simulink model "gm_sampleModel1492_sub"  (R2023a)
settings: Solver=VariableStepAuto  StartTime=0.0  StopTime=10.0  RelTol=1e-3
libraries: hdlsllib x2, simulink x1
settings Model: Creator=user1  LastModifiedBy=user1
settings OptimizationCC: BlockReduction=off  ConditionallyExecuteInputs=off
settings DebuggingCC: InheritedTsInSrcMsg=none

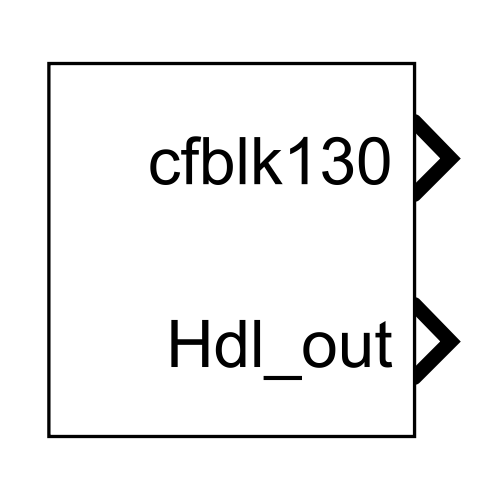
[thumbnail: Simulink's stored preview of the top-level diagram]
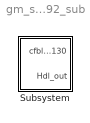
== system gm_sampleModel1492_sub ==
  Subsystem : Subsystem

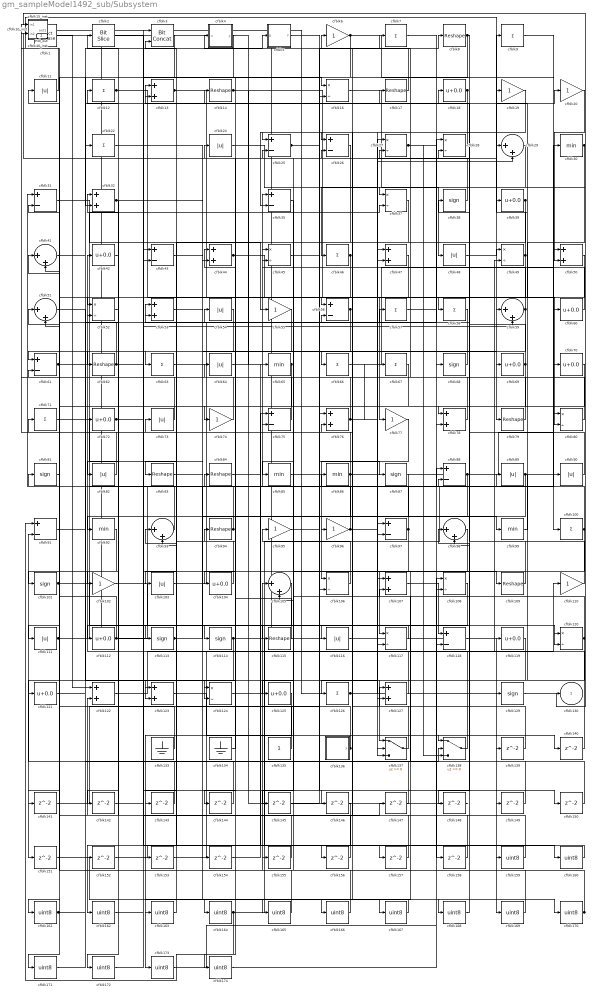
== system gm_sampleModel1492_sub/Subsystem ==
  cfblk1 : simulink/Logic and Bit Operations/Detect Decrease  vinit=0.0  OutDataTypeStr=uint8
      settings: LibrarySourceBlock=|
      | hdlsllib/Logic and Bit
      | Operations/Detect
      | Decrease
  cfblk{7,9,12,22,46,57..58,63,66..67,71,100,126} (13 alike) : Sum  Inputs=+  OutDataTypeStr=uint8
  cfblk{38,68,81,87,101,113..114,129} (8 alike) : Signum
  cfblk{6,19..20,55,74,77,95..96,102,110} (10 alike) : Gain  OutDataTypeStr=uint8
  cfblk{11,24,48,54,64,73,82,89..90,103,111,116} (12 alike) : Abs  OutDataTypeStr=uint8  SaturateOnIntegerOverflow=off
  cfblk{18,39,42,60,69..70,72,104,112,119,121,125} (12 alike) : Bias  Bias=0.0  SaturateOnIntegerOverflow=off
  cfblk{29,41,51,59,93,98,105} (7 alike) : Sum  Inputs=|++  OutDataTypeStr=uint8
  cfblk{16,27..28,37,45,49,52,80,106,108,117,120,124} (13 alike) : Product  Inputs=*/  OutDataTypeStr=uint8  RndMeth=Zero  SaturateOnIntegerOverflow=on
  cfblk{13,32,44,47,50,53,76,78,107,122..123,127} (12 alike) : Sum  OutDataTypeStr=uint8
  cfblk{8,14,17,62,79,83..84,94,109,115} (10 alike) : Reshape
  cfblk10_inst : Subsystem
  cfblk{25..26,31,35,43,56,61,75,88,91,97,118} (12 alike) : Sum  Inputs=+-  OutDataTypeStr=uint8
  cfblk133 : Ground
  cfblk134 : Ground
  cfblk135 : Constant  OutDataTypeStr=uint8  SampleTime=-1
  cfblk136 : Subsystem  mask(Counter Limited){uplimit=double(7), tsamp=double(-1)}
      mask prompts: uplimit "Simulink:masks:UpperLimit_MP"; tsamp "Simulink:masks:SampleTime_MP"
      mask help: Simulink:masks:CounterLimited_MD
      mask init:
      | nbits = double(8);
      | tsamp = double(-1);
      | uplimit = double(7);
  cfblk137 : Switch  OutDataTypeStr=uint8  SaturateOnIntegerOverflow=off  InputSameDT=off
  cfblk138 : Switch  OutDataTypeStr=uint8  SaturateOnIntegerOverflow=off  InputSameDT=off
  cfblk{139..158} (20 alike) : Delay  SampleTime=1
  cfblk{159..174} (16 alike) : DataTypeConversion  OutDataTypeStr=uint8  SaturateOnIntegerOverflow=off  RndMeth=Floor
  cfblk15_inst : Subsystem
  cfblk2 : hdlsllib/Logic and Bit Operations/Bit Slice  lidx=7  ridx=0
  cfblk3 : hdlsllib/Logic and Bit Operations/Bit Concat  numInputs=2
  cfblk{30,65,85..86,92,99} (6 alike) : MinMax  OutDataTypeStr=uint8
  cfblk4 : Subsystem  mask(Compare To Zero){relop=<=, OutDataTypeStr=uint8, ZeroCross=on}
      mask prompts: relop "Simulink:masks:Operator_MP"; OutDataTypeStr "Simulink:masks:OutputDataType_MP"; ZeroCross "Simulink:masks:EnableZerocrossingDetection_MP"
      mask help: Simulink:masks:CompareToZero_MD
      mask init:
      | OutDataTypeStr = 'uint8';
      | ZeroCross = 'on';
      | blkName = 'sampleModel1492_sub/Subsystem/cfblk4';
      | relop = '<=';
      | setValue = 'fixdt(0, 8)';
      mask TypeOptions relop: == | ~= | < | <= | >= | >
      mask TypeOptions OutDataTypeStr: Simulink:masks:uint8 | Simulink:masks:boolean
      mask Callback ZeroCross: sl('zeroCrossEnable', gcbh);
      mask Display: disp([relop,' 0'])
  cfblk40_inst : Subsystem
  cfblk5 : Subsystem  mask(Detect Fall Nonpositive){vinit=double(0), InputProcessing=Elements as channels (sample based), OutDataTypeStr=uint8}
      mask prompts: vinit "Simulink:masks:InitialCondition_MP"; InputProcessing "Simulink:masks:InputProcessing_MP"; OutDataTypeStr "Simulink:masks:OutputDataType_MP"
      mask help: Simulink:masks:DetectFallNonpositive_MD
      mask init:
      | InputProcessing = 'Elements as channels (sample based)';
      | OutDataTypeStr = 'uint8';
      | vinit = double(0);
      mask TypeOptions InputProcessing: Simulink:masks:ColumnsAsChannelsFrameBased | Simulink:masks:ElementsAsChannelsSampleBased
      mask TypeOptions OutDataTypeStr: Simulink:masks:uint8 | Simulink:masks:boolean
      mask Display: fprintf('U <= 0\n&  NOT\nU/z <= 0')
  cfblk130 : Outport  OutDataTypeStr=uint8  SampleTime=1  VectorParamsAs1DForOutWhenUnconnected=off
  Hdl_out : Outport  Port=2  OutDataTypeStr=uint8  SampleTime=1
  wires:
  cfblk1/1 -> cfblk122/1
  cfblk10_inst/1(out1) -> cfblk90/1
  cfblk100/1 -> cfblk81/1, cfblk35/1, cfblk117/1
  cfblk101/1 -> cfblk116/1, cfblk120/2
  cfblk102/1 -> cfblk114/1
  cfblk103/1 -> cfblk56/2
  cfblk104/1 -> cfblk73/1
  cfblk105/1 -> cfblk164/1
  cfblk106/1 -> cfblk95/1
  cfblk107/1 -> cfblk118/1
  cfblk108/1 -> cfblk172/1
  cfblk109/1 -> cfblk13/1
  cfblk11/1 -> cfblk79/1
  cfblk110/1 -> cfblk53/1
  cfblk111/1 -> cfblk84/1, cfblk37/2
  cfblk112/1 -> cfblk88/2, cfblk11/1
  cfblk113/1 -> cfblk88/1, Hdl_out/1
  cfblk114/1 -> cfblk160/1, cfblk123/2, cfblk151/1
  cfblk115/1 -> cfblk54/1
  cfblk116/1 -> cfblk107/1
  cfblk117/1 -> cfblk113/1
  cfblk118/1 -> cfblk169/1
  cfblk119/1 -> cfblk137/1
  cfblk12/1 -> cfblk80/2, cfblk16/1
  cfblk120/1 -> cfblk45/1, cfblk126/1
  cfblk121/1 -> cfblk5/1(U)
  cfblk122/1 -> cfblk110/1
  cfblk123/1 -> cfblk138/1
  cfblk124/1 -> cfblk140/1
  cfblk125/1 -> cfblk173/1
  cfblk126/1 -> cfblk47/2, cfblk6/1
  cfblk127/1 -> cfblk75/2
  cfblk129/1 -> cfblk10_inst/1(in1)
  cfblk13/1 -> cfblk158/1, cfblk117/2
  cfblk133/1 -> cfblk51/1
  cfblk134/1 -> cfblk44/1
  cfblk135/1 -> cfblk94/1
  cfblk136/1(y) -> cfblk24/1, cfblk13/2
  cfblk137/1 -> cfblk76/2
  cfblk138/1 -> cfblk42/1
  cfblk139/1 -> cfblk127/1
  cfblk14/1 -> cfblk60/1, cfblk65/1
  cfblk140/1 -> cfblk47/1
  cfblk141/1 -> cfblk16/2
  cfblk142/1 -> cfblk43/2
  cfblk143/1 -> cfblk91/2
  cfblk144/1 -> cfblk52/2
  cfblk145/1 -> cfblk76/1
  cfblk146/1 -> cfblk162/1
  cfblk147/1 -> cfblk53/2
  cfblk148/1 -> cfblk1/1
  cfblk149/1 -> cfblk107/2
  cfblk15_inst/1(out1) -> cfblk119/1
  cfblk150/1 -> cfblk93/1
  cfblk151/1 -> cfblk168/1
  cfblk152/1 -> cfblk159/1
  cfblk153/1 -> cfblk49/2
  cfblk154/1 -> cfblk75/1
  cfblk155/1 -> cfblk122/2
  cfblk156/1 -> cfblk32/1
  cfblk157/1 -> cfblk41/2
  cfblk158/1 -> cfblk2/1
  cfblk159/1 -> cfblk26/2
  cfblk16/1 -> cfblk48/1
  cfblk160/1 -> cfblk152/1
  cfblk161/1 -> cfblk18/1, cfblk138/2
  cfblk162/1 -> cfblk3/1
  cfblk163/1 -> cfblk3/2
  cfblk164/1 -> cfblk91/1, cfblk80/1
  cfblk165/1 -> cfblk105/1
  cfblk166/1 -> cfblk105/2
  cfblk167/1 -> cfblk163/1
  cfblk168/1 -> cfblk98/1
  cfblk169/1 -> cfblk98/2
  cfblk17/1 -> cfblk4/1(u)
  cfblk170/1 -> cfblk155/1, cfblk71/1
  cfblk171/1 -> cfblk22/1
  cfblk172/1 -> cfblk147/1
  cfblk173/1 -> cfblk108/1
  cfblk174/1 -> cfblk108/2
  cfblk18/1 -> cfblk35/2, cfblk166/1, cfblk137/3
  cfblk19/1 -> cfblk26/1
  cfblk2/1 -> cfblk109/1
  cfblk20/1 -> cfblk50/2
  cfblk22/1 -> cfblk170/1
  cfblk24/1 -> cfblk97/1
  cfblk25/1 -> cfblk87/1, cfblk58/1
  cfblk26/1 -> cfblk93/2
  cfblk27/1 -> cfblk68/1, cfblk138/3
  cfblk28/1 -> cfblk25/1
  cfblk29/1 -> cfblk46/1
  cfblk3/1 -> cfblk161/1
  cfblk30/1 -> cfblk59/1, cfblk37/1
  cfblk31/1 -> cfblk55/1
  cfblk32/1 -> cfblk44/2, cfblk112/1
  cfblk35/1 -> cfblk115/1
  cfblk37/1 -> cfblk145/1
  cfblk38/1 -> cfblk15_inst/2(in2)
  cfblk39/1 -> cfblk123/1, cfblk74/1
  cfblk4/1(y) -> cfblk32/2
  cfblk40_inst/1(out1) -> cfblk130/1
  cfblk41/1 -> cfblk17/1
  cfblk42/1 -> cfblk82/1
  cfblk43/1 -> cfblk69/1
  cfblk44/1 -> cfblk97/2, cfblk77/1
  cfblk45/1 -> cfblk8/1
  cfblk46/1 -> cfblk111/1, cfblk45/2, cfblk144/1
  cfblk47/1 -> cfblk63/1
  cfblk48/1 -> cfblk49/1
  cfblk49/1 -> cfblk118/2, cfblk9/1
  cfblk5/1(Y) -> cfblk150/1
  cfblk50/1 -> cfblk52/1
  cfblk51/1 -> cfblk127/2
  cfblk52/1 -> cfblk92/1
  cfblk53/1 -> cfblk99/1
  cfblk54/1 -> cfblk171/1
  cfblk55/1 -> cfblk143/1
  cfblk56/1 -> cfblk83/1, cfblk124/2
  cfblk57/1 -> cfblk120/1
  cfblk58/1 -> cfblk85/1
  cfblk59/1 -> cfblk78/1, cfblk56/1, cfblk25/2
  cfblk6/1 -> cfblk70/1, cfblk61/1
  cfblk60/1 -> cfblk39/1
  cfblk61/1 -> cfblk121/1, cfblk28/1
  cfblk62/1 -> cfblk14/1, cfblk10_inst/2(in2), cfblk149/1
  cfblk63/1 -> cfblk27/1
  cfblk64/1 -> cfblk157/1
  cfblk65/1 -> cfblk141/1, cfblk124/1
  cfblk66/1 -> cfblk30/1
  cfblk67/1 -> cfblk142/1
  cfblk68/1 -> cfblk62/1
  cfblk69/1 -> cfblk78/2, cfblk104/1, cfblk28/2, cfblk66/1
  cfblk7/1 -> cfblk139/1
  cfblk70/1 -> cfblk153/1
  cfblk71/1 -> cfblk154/1
  cfblk72/1 -> cfblk59/2, cfblk20/1, cfblk156/1
  cfblk73/1 -> cfblk41/1
  cfblk74/1 -> cfblk15_inst/1(in1)
  cfblk75/1 -> cfblk43/1
  cfblk76/1 -> cfblk31/2, cfblk29/2, cfblk67/1
  cfblk77/1 -> cfblk106/1
  cfblk78/1 -> cfblk64/1
  cfblk79/1 -> cfblk7/1
  cfblk8/1 -> cfblk174/1, cfblk148/1
  cfblk80/1 -> cfblk27/2
  cfblk81/1 -> cfblk51/2
  cfblk82/1 -> cfblk40_inst/1(in1)
  cfblk83/1 -> cfblk165/1
  cfblk84/1 -> cfblk146/1
  cfblk85/1 -> cfblk106/2
  cfblk86/1 -> cfblk40_inst/2(in2), cfblk102/1
  cfblk87/1 -> cfblk96/1
  cfblk88/1 -> cfblk50/1, cfblk103/1
  cfblk89/1 -> cfblk137/2, cfblk129/1
  cfblk9/1 -> cfblk100/1
  cfblk90/1 -> cfblk38/1
  cfblk91/1 -> cfblk57/1
  cfblk92/1 -> cfblk101/1
  cfblk93/1 -> cfblk12/1
  cfblk94/1 -> cfblk61/2, cfblk31/1
  cfblk95/1 -> cfblk89/1
  cfblk96/1 -> cfblk29/1, cfblk86/1
  cfblk97/1 -> cfblk72/1, cfblk125/1
  cfblk98/1 -> cfblk167/1
  cfblk99/1 -> cfblk19/1

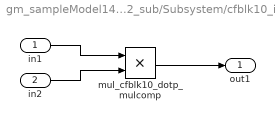
== system gm_sampleModel1492_sub/Subsystem/cfblk10_inst ==
  in1 : Inport  OutDataTypeStr=uint8  SampleTime=1
  in2 : Inport  Port=2  OutDataTypeStr=uint8  SampleTime=1
  mul_cfblk10_dotp_mulcomp : Product  Inputs=**  OutDataTypeStr=uint8  SampleTime=1
  out1 : Outport  OutDataTypeStr=uint8  SampleTime=1
  wires:
  in1/1 -> mul_cfblk10_dotp_mulcomp/1
  in2/1 -> mul_cfblk10_dotp_mulcomp/2
  mul_cfblk10_dotp_mulcomp/1 -> out1/1

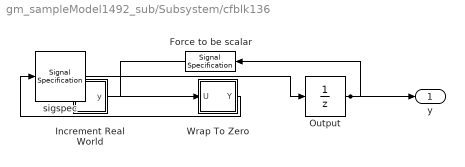
== system gm_sampleModel1492_sub/Subsystem/cfblk136 ==
  Force to be scalar : SignalSpecification  DisableCoverage=on  Dimensions=1
  Increment Real World : Subsystem  mask(Real World Value Increment){}
      mask help: Simulink:masks:RealWorldValueIncrement_MD
      mask Display: disp('V++')
  Output : UnitDelay  InitialCondition=0.0  SampleTime=tsamp  HasFrameUpgradeWarning=on
  Wrap To Zero : Subsystem  mask(Wrap To Zero){Threshold=double(7)}
      mask prompts: Threshold "Simulink:masks:Threshold_MP"
      mask help: Simulink:masks:WrapToZero_MD
  sigspec : SignalSpecification  OutDataTypeStr=uint8  Dimensions=1
  y : Outport  SampleTime=1
  wires:
  Force to be scalar/1 -> Increment Real World/1(u)
  Increment Real World/1(y) -> Wrap To Zero/1(U)
  Output/1 -> Force to be scalar/1, y/1
  Wrap To Zero/1(Y) -> sigspec/1
  sigspec/1 -> Output/1

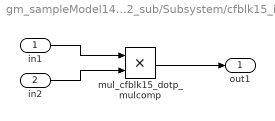
== system gm_sampleModel1492_sub/Subsystem/cfblk15_inst ==
  in1 : Inport  OutDataTypeStr=uint8  SampleTime=1
  in2 : Inport  Port=2  OutDataTypeStr=uint8  SampleTime=1
  mul_cfblk15_dotp_mulcomp : Product  Inputs=**  OutDataTypeStr=uint8  SampleTime=1
  out1 : Outport  OutDataTypeStr=uint8  SampleTime=1
  wires:
  in1/1 -> mul_cfblk15_dotp_mulcomp/1
  in2/1 -> mul_cfblk15_dotp_mulcomp/2
  mul_cfblk15_dotp_mulcomp/1 -> out1/1

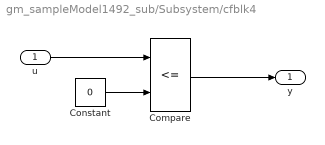
== system gm_sampleModel1492_sub/Subsystem/cfblk4 ==
  u : Inport  OutDataTypeStr=uint8  SampleTime=1
  Compare : RelationalOperator  Operator=<=  OutDataTypeStr=fixdt(0, 8)
  Constant : Constant  DisableCoverage=on  Value=0  OutDataTypeStr=Inherit: Inherit via back propagation  SampleTime=-1  PreserveConstantTs=on
  y : Outport  SampleTime=1
  wires:
  u/1 -> Compare/1
  Compare/1 -> y/1
  Constant/1 -> Compare/2

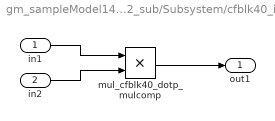
== system gm_sampleModel1492_sub/Subsystem/cfblk40_inst ==
  in1 : Inport  OutDataTypeStr=uint8  SampleTime=1
  in2 : Inport  Port=2  OutDataTypeStr=uint8  SampleTime=1
  mul_cfblk40_dotp_mulcomp : Product  Inputs=**  OutDataTypeStr=uint8  SampleTime=1
  out1 : Outport  OutDataTypeStr=uint8  SampleTime=1
  wires:
  in1/1 -> mul_cfblk40_dotp_mulcomp/1
  in2/1 -> mul_cfblk40_dotp_mulcomp/2
  mul_cfblk40_dotp_mulcomp/1 -> out1/1

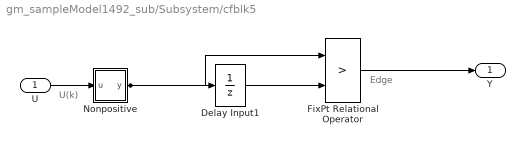
== system gm_sampleModel1492_sub/Subsystem/cfblk5 ==
  note: U(k)
  note: Edge
  U : Inport  OutDataTypeStr=uint8  SampleTime=1
  Delay Input1 : UnitDelay  Description=Store in Global RAM  DisableCoverage=on  InitialCondition=vinit  SampleTime=-1  HasFrameUpgradeWarning=on
  FixPt Relational Operator : RelationalOperator  Operator=>  OutDataTypeStr=fixdt(0, 8)  ZeroCross=off  InputSameDT=off
  Nonpositive : Subsystem  mask(Compare To Zero){relop=<=, OutDataTypeStr=boolean, ZeroCross=off}
      mask prompts: relop "Simulink:masks:Operator_MP"; OutDataTypeStr "Simulink:masks:OutputDataType_MP"; ZeroCross "Simulink:masks:EnableZerocrossingDetection_MP"
      mask help: Simulink:masks:CompareToZero_MD
      mask init:
      | OutDataTypeStr = 'boolean';
      | ZeroCross = 'off';
      | blkName = 'sampleModel1492_sub/Subsystem/cfblk5/Nonpositive';
      | relop = '<=';
      | setValue = 'boolean';
      mask TypeOptions relop: == | ~= | < | <= | >= | >
      mask TypeOptions OutDataTypeStr: Simulink:masks:uint8 | Simulink:masks:boolean
      mask Callback ZeroCross: sl('zeroCrossEnable', gcbh);
      mask Display: disp([relop,' 0'])
  Y : Outport  SampleTime=1
  wires:
  U/1 -> Nonpositive/1(u)
  Delay Input1/1 -> FixPt Relational Operator/2
  FixPt Relational Operator/1 -> Y/1
  Nonpositive/1(y) -> FixPt Relational Operator/1, Delay Input1/1

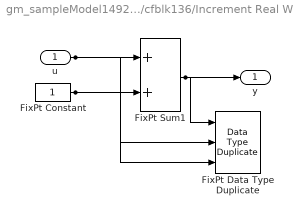
== system gm_sampleModel1492_sub/Subsystem/cfblk136/Increment Real World ==
  u : Inport  OutDataTypeStr=uint8  SampleTime=1
  FixPt Constant : Constant  DisableCoverage=on  OutDataTypeStr=Inherit: Inherit via back propagation  SampleTime=-1
  FixPt Data Type Duplicate : DataTypeDuplicate  DisableCoverage=on  NumInputPorts=3
  FixPt Sum1 : Sum  InputSameDT=on  OutDataTypeStr=Inherit: Inherit via back propagation  LockScale=on
  y : Outport  SampleTime=1
  wires:
  u/1 -> FixPt Sum1/1, FixPt Data Type Duplicate/2
  FixPt Constant/1 -> FixPt Sum1/2, FixPt Data Type Duplicate/3
  FixPt Sum1/1 -> FixPt Data Type Duplicate/1, y/1

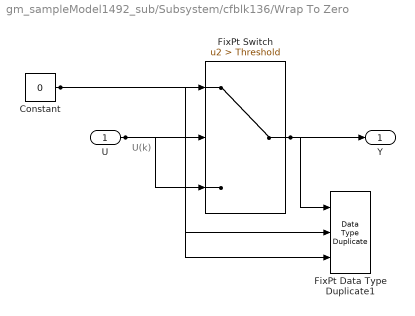
== system gm_sampleModel1492_sub/Subsystem/cfblk136/Wrap To Zero ==
  note: U(k)
  U : Inport  OutDataTypeStr=uint8  SampleTime=1
  Constant : Constant  DisableCoverage=on  Value=0  OutDataTypeStr=Inherit: Inherit via back propagation  SampleTime=-1
  FixPt Data Type Duplicate1 : DataTypeDuplicate  DisableCoverage=on  NumInputPorts=3
  FixPt Switch : Switch  Criteria=u2 > Threshold  Threshold=Threshold  OutDataTypeStr=Inherit: Inherit via back propagation  ZeroCross=off  SaturateOnIntegerOverflow=off  InputSameDT=off
  Y : Outport  SampleTime=1
  wires:
  U/1 -> FixPt Switch/3, FixPt Switch/2, FixPt Data Type Duplicate1/2
  Constant/1 -> FixPt Switch/1, FixPt Data Type Duplicate1/3
  FixPt Switch/1 -> FixPt Data Type Duplicate1/1, Y/1

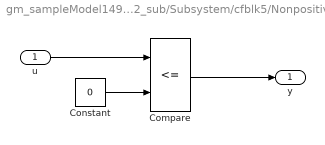
== system gm_sampleModel1492_sub/Subsystem/cfblk5/Nonpositive ==
  u : Inport  OutDataTypeStr=uint8  SampleTime=1
  Compare : RelationalOperator  Operator=<=  OutDataTypeStr=boolean  ZeroCross=off
  Constant : Constant  DisableCoverage=on  Value=0  OutDataTypeStr=Inherit: Inherit via back propagation  SampleTime=-1  PreserveConstantTs=on
  y : Outport  SampleTime=1
  wires:
  u/1 -> Compare/1
  Compare/1 -> y/1
  Constant/1 -> Compare/2
